simulink library "softmpc"  (R2014a)
settings: Solver=ode45  StartTime=0.0  StopTime=10.0  RelTol=1e-3
values from neighbouring files (symbols this model uses):
  bd = [kron(ones(T,1),eye(n))]    [buildmatrices.m]
  bx = [A; zeros(ellef+(T-1)*n,n)]    [buildmatrices.m]
  C = [kron(eye(T),[-B eye(n)]) + kron([zeros(1,T); eye(T-1) zeros(T-1,1)],[zeros(n,m) -A]); zeros(ellef,m+(T-1)*(m+n)) Ef]    [buildmatrices.m]
  Ef_block = zeros(2*n,1)    [buildmatrices.m]
  g = [r; repmat([q;r],T-1,1); qf]    [buildmatrices.m]
  gt = kron(ones(T,1),[zeros(1,n); -2*Q])    [buildmatrices.m]
  H = blkdiag(R,kron(eye(T-1),blkdiag(Q,R)),Qf)    [buildmatrices.m]
  hc = [repmat(f,T,1);ff]    [buildmatrices.m]
  hcs = [repmat(fs,T,1)]    [buildmatrices.m]
  hx = [-Fx; zeros((T-1)*ell + ellf,n)]    [buildmatrices.m]
  hxs = [-Fxs; zeros((T-1)*ells,n)]    [buildmatrices.m]
  P = blkdiag(Fu,kron(eye(T-1),[Fx Fu]),Ff)    [buildmatrices.m]    (also in test_ks_centre.m = [1 -1.5]')
  Ps = blkdiag(Fus,kron(eye(T-1),[Fxs Fus]))    [buildmatrices.m]
undefined symbols (not defined in the file or in its folder): A, B, Fu, Fus, Fx, Fxf, Fxs, hp, hps, Q, Qf, R
undefined symbols (not defined in the file): Ed, ef, Ef, f, ff, Fp, Fpf, Fps, fs, q, qf, r
settings Model: Creator=aeagr  LastModifiedBy=aeagr

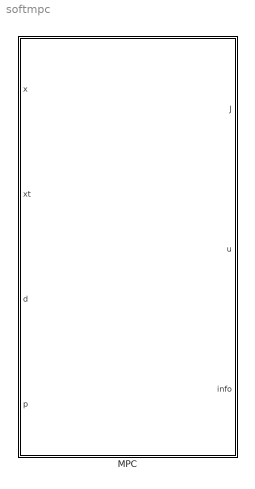
== system softmpc ==
  MPC : Subsystem  TreatAsAtomicUnit=on  mask{A=A, B=B, T=5, dt=-1, Q=Q, R=R, Qf=Qf, qv=q, rv=r, qfv=qf, Fx=Fx, Fu=Fu, Fp=Fp, f=f, Fxs=Fxs, Fus=Fus, Fps=Fps, fs=fs, Fxf=Fxf, Fpf=Fpf, ff=ff, Ef=Ef, Ed=Ed, e=ef, consAllBox=on, numNewton=5, kappa=0.005}
      mask prompts: T "Horizon length T"; dt "Time step"; qv "q"; rv "r"; qfv "qf"; e "ef"; consAllBox "Box constraints"; numNewton "Number of Newton Iterations"; kappa "Barrier weight kappa"
      mask init:
      | % build the big matrices
      | [H,g,gt,P,hx,hc,C,bx,bd,Ps,hxs,hcs,Ef_block,Ed_block,ef_block,hp,hps] = buildmatrices(A,B,Q,R,qv,rv,Qf,qfv,T,Fx,Fu,f,Fxs,Fus,fs,Fxf,ff,Ef,e,Ed,Fp,Fps,Fpf);
      | 
      | % options
      | opts=[];
      | disp(consAllBox)
      | if consAllBox,
      |     opts(1)=1; % 1 = assume diagonal Phi when solving
      | else
      |     opts(1)=0;
      | end
      | opts(2)=numNewton; % Newton iterations
      | opts(3)=1; % 1 = use soft constraints
      | opts(4)=0; % 1 = checking on
      | opts(7)=kappa; % tuning of barrier weight kappa

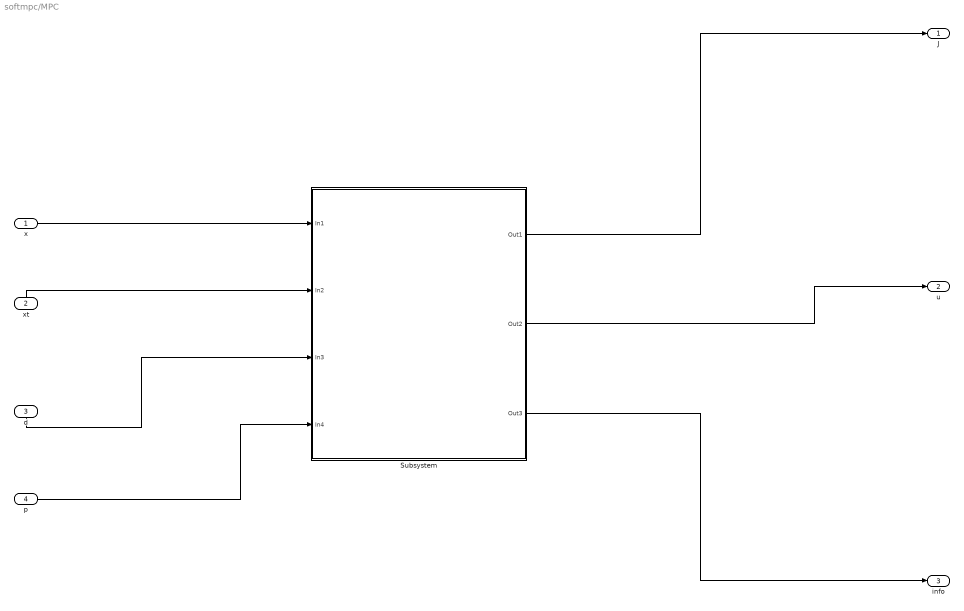
== system softmpc/MPC ==
  x : Inport
  xt : Inport  Port=2
  d : Inport  Port=3
  p : Inport  Port=4
  Subsystem : Subsystem  TreatAsAtomicUnit=on  SystemSampleTime=dt
  J : Outport
  u : Outport  Port=2
  info : Outport  Port=3
  wires:
  Subsystem/3(Out3) -> info/1
  Subsystem/2(Out2) -> u/1
  Subsystem/1(Out1) -> J/1
  p/1 -> Subsystem/4(In4)
  d/1 -> Subsystem/3(In3)
  xt/1 -> Subsystem/2(In2)
  x/1 -> Subsystem/1(In1)

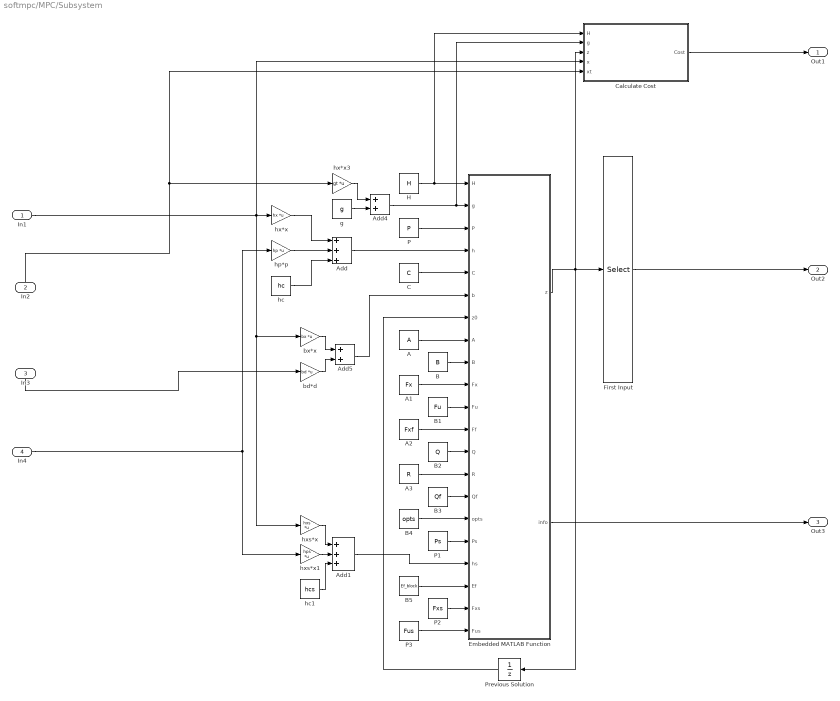
== system softmpc/MPC/Subsystem ==
  In1 : Inport
  In2 : Inport  Port=2
  In3 : Inport  Port=3
  In4 : Inport  Port=4
  A : Constant  Value=A
  A1 : Constant  Value=Fx
  A2 : Constant  Value=Fxf
  A3 : Constant  Value=R
  Add : Sum  Inputs=+++
  Add1 : Sum  Inputs=+++
  Add4 : Sum
  Add5 : Sum
  B : Constant  Value=B
  B1 : Constant  Value=Fu
  B2 : Constant  Value=Q
  B3 : Constant  Value=Qf
  B4 : Constant  Value=opts
  B5 : Constant  Value=Ef_block
  C : Constant  Value=C
  Calculate Cost : Subsystem
  Embedded MATLAB Function : MATLAB Function  TreatAsAtomicUnit=on
      settings: RTWFileNameOpts=Use subsystem name
  First Input : Selector  InputPortWidth=size(H,1)  Indices=1:size(B,2)
  H : Constant  Value=H
  P : Constant  Value=P
  P1 : Constant  Value=Ps
  P2 : Constant  Value=Fxs
  P3 : Constant  Value=Fus
  Previous Solution : UnitDelay  SampleTime=-1
  bd*d : Gain  Gain=bd  Multiplication=Matrix(K*u)
  bx*x : Gain  Gain=bx  Multiplication=Matrix(K*u)
  g : Constant  Value=g
  hc : Constant  Value=hc
  hc1 : Constant  Value=hcs
  hp*p : Gain  Gain=hp  Multiplication=Matrix(K*u)
  hx*x : Gain  Gain=hx  Multiplication=Matrix(K*u)
  hx*x3 : Gain  Gain=gt  Multiplication=Matrix(K*u)
  hxs*x : Gain  Gain=hxs  Multiplication=Matrix(K*u)
  hxs*x1 : Gain  Gain=hps  Multiplication=Matrix(K*u)
  Out1 : Outport
  Out2 : Outport  Port=2
  Out3 : Outport  Port=3
  wires:
  Calculate Cost/1(Cost) -> Out1/1
  B2/1 -> Embedded MATLAB Function/13(Q)
  B4/1 -> Embedded MATLAB Function/16(opts)
  Add5/1 -> Embedded MATLAB Function/6(b)
  bd*d/1 -> Add5/2
  hc/1 -> Add/3
  P1/1 -> Embedded MATLAB Function/17(Ps)
  B5/1 -> Embedded MATLAB Function/19(Ef)
  P3/1 -> Embedded MATLAB Function/21(Fus)
  hc1/1 -> Add1/3
  hxs*x1/1 -> Add1/2
  hp*p/1 -> Add/2
  hx*x3/1 -> Add4/1
  B1/1 -> Embedded MATLAB Function/11(Fu)
  Add4/1 -> Calculate Cost/2(g), Embedded MATLAB Function/2(g)
  hxs*x/1 -> Add1/1
  bx*x/1 -> Add5/1
  A1/1 -> Embedded MATLAB Function/10(Fx)
  Add1/1 -> Embedded MATLAB Function/18(hs)
  In4/1 -> hxs*x1/1, hp*p/1
  Embedded MATLAB Function/2(info) -> Out3/1
  P2/1 -> Embedded MATLAB Function/20(Fxs)
  g/1 -> Add4/2
  A2/1 -> Embedded MATLAB Function/12(Ff)
  In1/1 -> hx*x/1, hxs*x/1, bx*x/1, Calculate Cost/4(x)
  In3/1 -> bd*d/1
  In2/1 -> hx*x3/1, Calculate Cost/5(xt)
  First Input/1 -> Out2/1
  A/1 -> Embedded MATLAB Function/8(A)
  B3/1 -> Embedded MATLAB Function/15(Qf)
  C/1 -> Embedded MATLAB Function/5(C)
  P/1 -> Embedded MATLAB Function/3(P)
  A3/1 -> Embedded MATLAB Function/14(R)
  Add/1 -> Embedded MATLAB Function/4(h)
  hx*x/1 -> Add/1
  B/1 -> Embedded MATLAB Function/9(B)
  Previous Solution/1 -> Embedded MATLAB Function/7(z0)
  Embedded MATLAB Function/1(z) -> Calculate Cost/3(z), First Input/1, Previous Solution/1
  H/1 -> Calculate Cost/1(H), Embedded MATLAB Function/1(H)

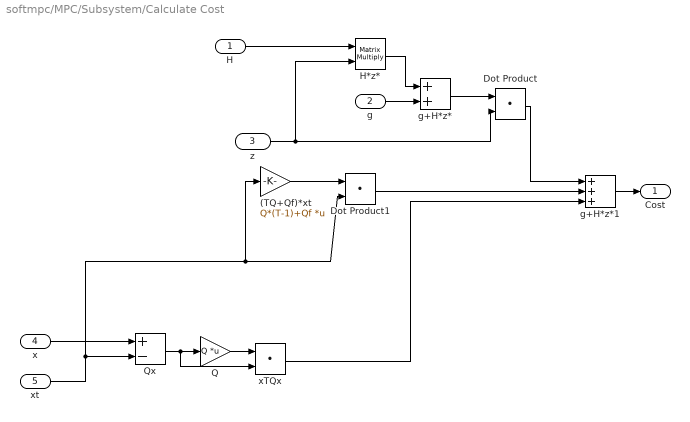
== system softmpc/MPC/Subsystem/Calculate Cost ==
  H : Inport
  g : Inport  Port=2
  z : Inport  Port=3
  x : Inport  Port=4
  xt : Inport  Port=5
  (TQ+Qf)*xt : Gain  Gain=Q*(T-1)+Qf  Multiplication=Matrix(K*u)
  Dot Product : DotProduct  InputSameDT=on  OutDataTypeStr=Inherit: Inherit via internal rule
  Dot Product1 : DotProduct  InputSameDT=on  OutDataTypeStr=Inherit: Inherit via internal rule
  H*z* : Product  Multiplication=Matrix(*)  RndMeth=Zero
  Q : Gain  Gain=Q  Multiplication=Matrix(K*u)
  Qx : Sum  Inputs=+-
  g+H*z* : Sum
  g+H*z*1 : Sum  Inputs=+++
  xTQx : DotProduct  InputSameDT=on  OutDataTypeStr=Inherit: Inherit via internal rule
  Cost : Outport
  wires:
  g+H*z*1/1 -> Cost/1
  xt/1 -> Dot Product1/2, (TQ+Qf)*xt/1, Qx/2
  x/1 -> Qx/1
  z/1 -> Dot Product/2, H*z*/2
  g/1 -> g+H*z*/2
  H/1 -> H*z*/1
  xTQx/1 -> g+H*z*1/3
  Q/1 -> xTQx/1
  Qx/1 -> xTQx/2, Q/1
  Dot Product1/1 -> g+H*z*1/2
  Dot Product/1 -> g+H*z*1/1
  (TQ+Qf)*xt/1 -> Dot Product1/1
  g+H*z*/1 -> Dot Product/1
  H*z*/1 -> g+H*z*/1

== matlab function softmpc/MPC/Subsystem/Embedded MATLAB Function ==
  data: H input; z output; g input; P input; h input; C input; b input size=size(C,1); z0 input; A input; B input; Fx input; Fu input; Ff input; Q input; R input; Qf input; info output; opts input; Ps input; hs input; Ef input; Fxs input; Fus input
function [z,info] = mpcsolve_simk(H,g,P,h,C,b,z0,A,B,Fx,Fu,Ff,Q,R,Qf,opts,Ps,hs,Ef,Fxs,Fus)
%#codegen

% just call to the Matlab version
[z,info] = mpcsolve(H,g,P,h,C,b,z0,A,B,Fx,Fu,Ff,Q,R,Qf,opts,Ps,hs,Ef,Fxs,Fus);
